simulink model "Gate_Harness"  (R2022b)
settings: Solver=VariableStepAuto  StartTime=0.0  StopTime=80.0  RelTol=1e-3
(part 1 of 2)
settings Model: Creator=chiar  LastModifiedBy=chiar
settings ConfigComp: CovEnable=on  RecordCoverage=on  CovModelRefEnable=on

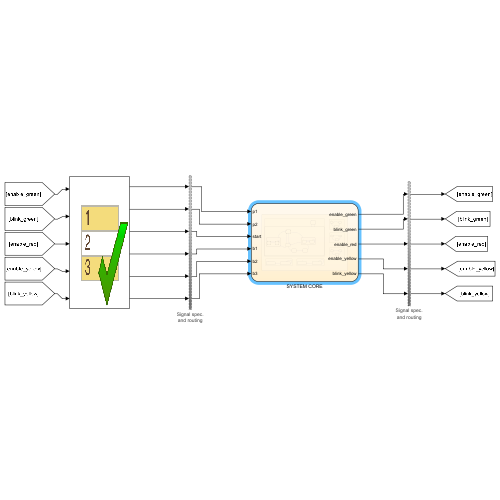
[thumbnail: Simulink's stored preview of the top-level diagram]
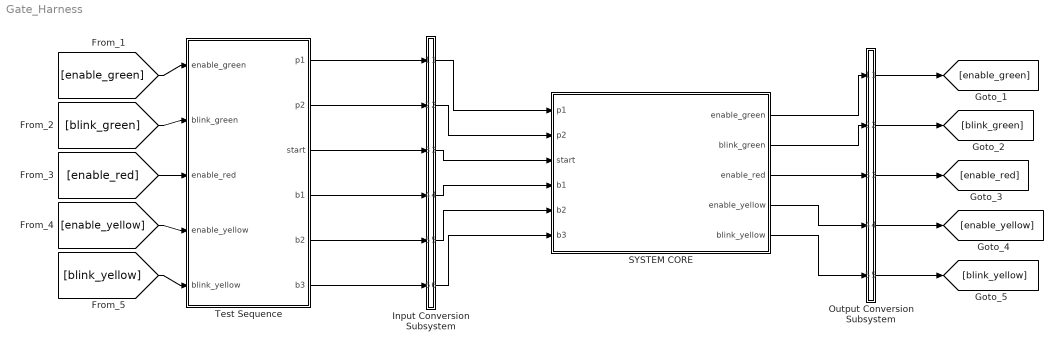
== system Gate_Harness ==
  Input Conversion Subsystem : Subsystem  Tag=__SLT_ICS__  Description=|
      | Signal spec.
      | and routing
      settings: AttributesFormatString=%<Description>
  Output Conversion Subsystem : Subsystem  Tag=__SLT_OCS__  Description=|
      | Signal spec.
      | and routing
      settings: AttributesFormatString=%<Description>
  SYSTEM CORE : Stateflow chart  TreatAsAtomicUnit=on
  Test Sequence : Test Sequence  TreatAsAtomicUnit=on
  wires:
  Test Sequence/1(p1) -> Input Conversion Subsystem/1(Inport_1)
  Test Sequence/2(p2) -> Input Conversion Subsystem/2(Inport_2)
  Test Sequence/3(start) -> Input Conversion Subsystem/3(Inport_3)
  Test Sequence/4(b1) -> Input Conversion Subsystem/4(Inport_4)
  Test Sequence/5(b2) -> Input Conversion Subsystem/5(Inport_5)
  Test Sequence/6(b3) -> Input Conversion Subsystem/6(Inport_6)
  [enable_green] -> Test Sequence/1(enable_green)
  [blink_green] -> Test Sequence/2(blink_green)
  [enable_red] -> Test Sequence/3(enable_red)
  [enable_yellow] -> Test Sequence/4(enable_yellow)
  [blink_yellow] -> Test Sequence/5(blink_yellow)
  Output Conversion Subsystem/1(Outport_1) -> [enable_green]
  Output Conversion Subsystem/2(Outport_2) -> [blink_green]
  Output Conversion Subsystem/3(Outport_3) -> [enable_red]
  Output Conversion Subsystem/4(Outport_4) -> [enable_yellow]
  Output Conversion Subsystem/5(Outport_5) -> [blink_yellow]
  Input Conversion Subsystem/1(Outport_1) -> SYSTEM CORE/1(p1)
  Input Conversion Subsystem/2(Outport_2) -> SYSTEM CORE/2(p2)
  Input Conversion Subsystem/3(Outport_3) -> SYSTEM CORE/3(start)
  Input Conversion Subsystem/4(Outport_4) -> SYSTEM CORE/4(b1)
  Input Conversion Subsystem/5(Outport_5) -> SYSTEM CORE/5(b2)
  Input Conversion Subsystem/6(Outport_6) -> SYSTEM CORE/6(b3)
  SYSTEM CORE/1(enable_green) -> Output Conversion Subsystem/1(Inport_1)
  SYSTEM CORE/2(blink_green) -> Output Conversion Subsystem/2(Inport_2)
  SYSTEM CORE/3(enable_red) -> Output Conversion Subsystem/3(Inport_3)
  SYSTEM CORE/4(enable_yellow) -> Output Conversion Subsystem/4(Inport_4)
  SYSTEM CORE/5(blink_yellow) -> Output Conversion Subsystem/5(Inport_5)

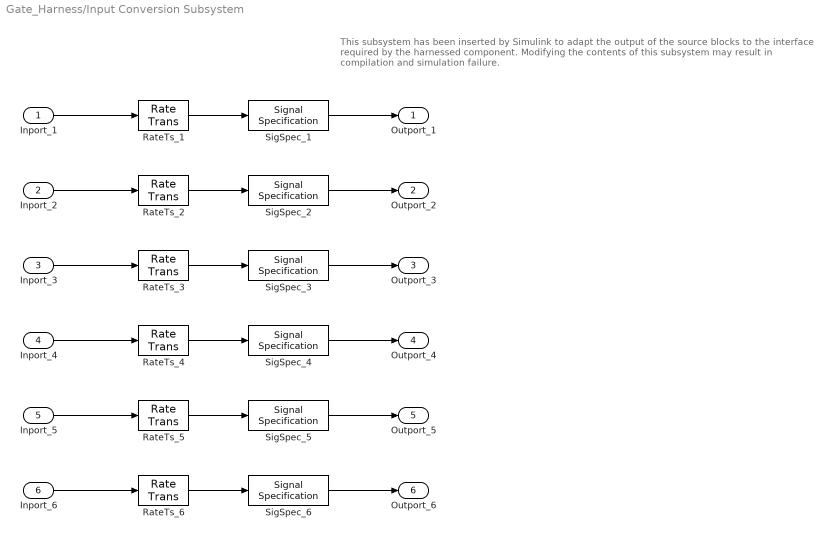
== system Gate_Harness/Input Conversion Subsystem ==
  note: This subsystem has been inserted by Simulink to adapt the output of the source blocks to the interface required by the harnessed component.
      |  Modifying the contents of this subsystem may result in compilation and simulation failure.
  Inport_1 : Inport
  Inport_2 : Inport  Port=2
  Inport_3 : Inport  Port=3
  Inport_4 : Inport  Port=4
  Inport_5 : Inport  Port=5
  Inport_6 : Inport  Port=6
  RateTs_{1..6} (6 alike) : RateTransition  OutPortSampleTime=[-1, 0]
  SigSpec_{1..6} (6 alike) : SignalSpecification  OutDataTypeStr=boolean  Dimensions=[1]  SampleTime=[-1, 0]
  Outport_1 : Outport
  Outport_2 : Outport  Port=2
  Outport_3 : Outport  Port=3
  Outport_4 : Outport  Port=4
  Outport_5 : Outport  Port=5
  Outport_6 : Outport  Port=6
  wires:
  SigSpec_1/1 -> Outport_1/1
  RateTs_1/1 -> SigSpec_1/1
  Inport_1/1 -> RateTs_1/1
  SigSpec_2/1 -> Outport_2/1
  RateTs_2/1 -> SigSpec_2/1
  Inport_2/1 -> RateTs_2/1
  SigSpec_3/1 -> Outport_3/1
  RateTs_3/1 -> SigSpec_3/1
  Inport_3/1 -> RateTs_3/1
  SigSpec_4/1 -> Outport_4/1
  RateTs_4/1 -> SigSpec_4/1
  Inport_4/1 -> RateTs_4/1
  SigSpec_5/1 -> Outport_5/1
  RateTs_5/1 -> SigSpec_5/1
  Inport_5/1 -> RateTs_5/1
  SigSpec_6/1 -> Outport_6/1
  RateTs_6/1 -> SigSpec_6/1
  Inport_6/1 -> RateTs_6/1

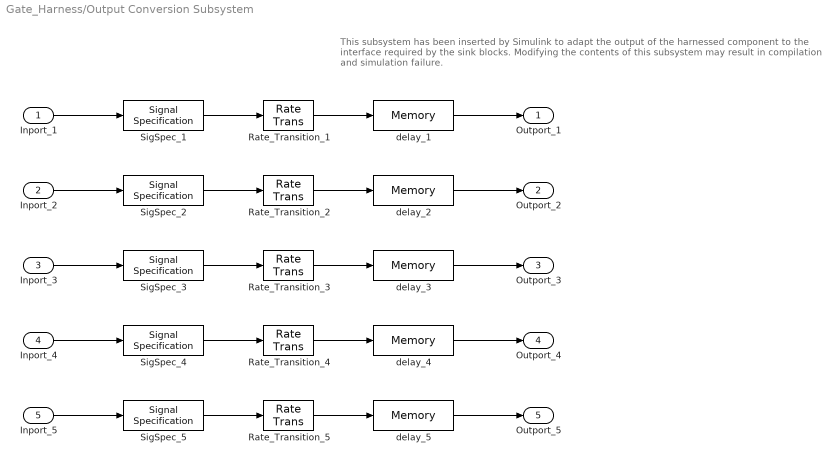
== system Gate_Harness/Output Conversion Subsystem ==
  note: This subsystem has been inserted by Simulink to adapt the output of the harnessed component to the interface required by the sink blocks.
      |  Modifying the contents of this subsystem may result in compilation and simulation failure.
  Inport_1 : Inport
  Inport_2 : Inport  Port=2
  Inport_3 : Inport  Port=3
  Inport_4 : Inport  Port=4
  Inport_5 : Inport  Port=5
  Rate_Transition_{1..5} (5 alike) : RateTransition  OutPortSampleTimeOpt=Inherit
  SigSpec_{1..5} (5 alike) : SignalSpecification  OutDataTypeStr=boolean  Dimensions=[1]
  delay_{1..5} (5 alike) : Memory
  Outport_1 : Outport
  Outport_2 : Outport  Port=2
  Outport_3 : Outport  Port=3
  Outport_4 : Outport  Port=4
  Outport_5 : Outport  Port=5
  wires:
  Inport_1/1 -> SigSpec_1/1
  SigSpec_1/1 -> Rate_Transition_1/1
  Rate_Transition_1/1 -> delay_1/1
  delay_1/1 -> Outport_1/1
  Inport_2/1 -> SigSpec_2/1
  SigSpec_2/1 -> Rate_Transition_2/1
  Rate_Transition_2/1 -> delay_2/1
  delay_2/1 -> Outport_2/1
  Inport_3/1 -> SigSpec_3/1
  SigSpec_3/1 -> Rate_Transition_3/1
  Rate_Transition_3/1 -> delay_3/1
  delay_3/1 -> Outport_3/1
  Inport_4/1 -> SigSpec_4/1
  SigSpec_4/1 -> Rate_Transition_4/1
  Rate_Transition_4/1 -> delay_4/1
  delay_4/1 -> Outport_4/1
  Inport_5/1 -> SigSpec_5/1
  SigSpec_5/1 -> Rate_Transition_5/1
  Rate_Transition_5/1 -> delay_5/1
  delay_5/1 -> Outport_5/1

== stateflow chart Gate_Harness/SYSTEM CORE ==
  state SYSTEM
    state GATE [parallel]
      settings: executionOrder=3
      state INACTIVE
        en:
        enable_green = OFF;
        enable_yellow = OFF;
        enable_red = OFF;
        blink_green = OFF;
        blink_yellow = OFF;
      state ACTIVE
        state IS_OPENING
          en:
          enable_red = OFF;
          enable_yellow=OFF;
          enable_green=OFF;
          blink_green = OFF;
          blink_yellow = ON;
        state OPEN
          state GREEN_BLK_OFF
            en:
            enable_green = ON;
            enable_red = ON;
            enable_yellow = ON;
            blink_green = OFF;
            blink_yellow = OFF;
          state GREEN_BLK_ON
            en:
            enable_green = OFF;
            enable_red = OFF;
            enable_yellow = OFF;
            blink_green = ON;
            blink_yellow = OFF;
          (default) -> SYSTEM.GATE.ACTIVE.OPEN.GREEN_BLK_OFF
          SYSTEM.GATE.ACTIVE.OPEN.GREEN_BLK_ON -> SYSTEM.GATE.ACTIVE.OPEN.GREEN_BLK_ON [order 2] : [b1_pressed & (p1 == OFF)]
          SYSTEM.GATE.ACTIVE.OPEN.GREEN_BLK_OFF -> SYSTEM.GATE.ACTIVE.OPEN.GREEN_BLK_ON : [b1_pressed & (p1 == OFF)]
          SYSTEM.GATE.ACTIVE.OPEN.GREEN_BLK_ON -> SYSTEM.GATE.ACTIVE.OPEN.GREEN_BLK_OFF [order 1] : [after(GREENDUR, sec) | (p1 == ON)]
        state CLOSE
          state GREEN_BLK_OFF
            en:
            enable_green = OFF;
            enable_red = OFF;
            enable_yellow = OFF;
            blink_green = OFF;
            blink_yellow = OFF;
          state GREEN_BLK_ON
            en:
            enable_green = OFF;
            enable_red = OFF;
            enable_yellow = OFF;
            blink_green = ON;
            blink_yellow = OFF;
          (default) -> SYSTEM.GATE.ACTIVE.CLOSE.GREEN_BLK_OFF
          SYSTEM.GATE.ACTIVE.CLOSE.GREEN_BLK_ON -> SYSTEM.GATE.ACTIVE.CLOSE.GREEN_BLK_ON [order 2] : [b1_pressed & (p1 == OFF)]
          SYSTEM.GATE.ACTIVE.CLOSE.GREEN_BLK_OFF -> SYSTEM.GATE.ACTIVE.CLOSE.GREEN_BLK_ON : [b1_pressed & (p1 == OFF)]
          SYSTEM.GATE.ACTIVE.CLOSE.GREEN_BLK_ON -> SYSTEM.GATE.ACTIVE.CLOSE.GREEN_BLK_OFF [order 1] : [after(GREENDUR, sec) | (p1 == ON)]
        state IS_CLOSING
          en:
          enable_red = OFF;
          enable_yellow=OFF;
          enable_green=OFF;
          blink_green = OFF;
          blink_yellow = ON;
        note: Per i sensori stiamo usando la logica negata.
        state STOP_SYSTEM
          en:
          enable_red = OFF;
          enable_yellow=OFF;
          enable_green=OFF;
          blink_green = OFF;
          blink_yellow = OFF;
        state ERROR_STATE
          en:
          enable_red = ON;
          enable_yellow=OFF;
          enable_green=OFF;
          blink_green = OFF;
          blink_yellow = OFF;
        IS_OPENING -> OPEN [order 2] : after(working_time, sec)
        CLOSE -> IS_OPENING : [b1_pressed & (p1 == ON)]
        IS_CLOSING -> IS_OPENING [order 1] : [b1_pressed | (p1 == OFF)]
        IS_OPENING -> IS_CLOSING [order 1] : [b1_pressed & (p1 == ON)]
        IS_CLOSING -> CLOSE [order 2] : [(p2 == OFF)]
        (default) -> IS_CLOSING
        ERROR_STATE -> CLOSE : [p2 == OFF]
        OPEN -> IS_CLOSING : [(b1_pressed & p1 == ON) | duration(p1 == ON) >= closing_time]
        IS_CLOSING -> STOP_SYSTEM [order 3] : [after(working_time, sec) & (p2 == ON)]
        STOP_SYSTEM -> ERROR_STATE : after(WAITING_TIME,sec)
      (default) -> INACTIVE
      INACTIVE -> ACTIVE : [start == ON]
      ACTIVE -> INACTIVE : [start == OFF]
    state B1 [parallel]
      settings: executionOrder=6
      state RELEASED
      state PRESSED
      state LONG_PRESSED
        send(b1_pressed)
      (default) -> SYSTEM.B1.RELEASED
      SYSTEM.B1.RELEASED -> SYSTEM.B1.PRESSED : [b1==ON]
      SYSTEM.B1.LONG_PRESSED -> SYSTEM.B1.RELEASED : [b1 == OFF]
      SYSTEM.B1.PRESSED -> SYSTEM.B1.LONG_PRESSED : [b1 == OFF]
    state B2 [parallel]
      settings: executionOrder=5
      state RELEASED
      state PRESSED
      state LONG_PRESSED
        send(b2_pressed)
      (default) -> SYSTEM.B2.RELEASED
      SYSTEM.B2.RELEASED -> SYSTEM.B2.PRESSED : [b2==ON]
      SYSTEM.B2.LONG_PRESSED -> SYSTEM.B2.RELEASED : [b2 == OFF]
      SYSTEM.B2.PRESSED -> SYSTEM.B2.LONG_PRESSED : [b2 == OFF]
    state B3 [parallel]
      settings: executionOrder=4
      state RELEASED
      state PRESSED
      state LONG_PRESSED
        send(b3_pressed)
      (default) -> SYSTEM.B3.RELEASED
      SYSTEM.B3.RELEASED -> SYSTEM.B3.PRESSED : [b3==ON]
      SYSTEM.B3.LONG_PRESSED -> SYSTEM.B3.RELEASED : [b3 == OFF]
      SYSTEM.B3.PRESSED -> SYSTEM.B3.LONG_PRESSED : [b3 == OFF]
    state WORKING_TIME [parallel]
      settings: executionOrder=1
      state WORKING_TIME_RESET
        en:
        working_time = 10;
      state WORKING_TIME_INC
        en:
        working_time = mod(working_time, MAX) + INCREMENT;
      WORKING_TIME_INC -> WORKING_TIME_INC : [b3_pressed & p2 == OFF]
      (default) -> WORKING_TIME_RESET
      WORKING_TIME_RESET -> WORKING_TIME_INC : [b3_pressed & p2 == OFF]
    state CLOSING_TIME [parallel]
      settings: executionOrder=2
      state CLOSING_TIME_RESET
        en:
        closing_time = 10;
      state CLOSING_TIME_INC
        en:
        closing_time = mod(closing_time, MAX) + INCREMENT;
      CLOSING_TIME_INC -> CLOSING_TIME_INC : [b2_pressed & p2 == OFF]
      (default) -> CLOSING_TIME_RESET
      CLOSING_TIME_RESET -> CLOSING_TIME_INC : [b2_pressed & p2 == OFF]
  data: GREENDUR constant double =30; WAITING_TIME constant double =10; ON constant boolean =1; OFF constant boolean =0; working_time local double =10; INCREMENT constant double =10; MAX constant double =120; closing_time local double =10; p1 input boolean; p2 input boolean; start input boolean; enable_green output boolean; blink_green output boolean; enable_red output boolean; enable_yellow output boolean; blink_yellow output boolean; b1 input boolean; b2 input boolean; b3 input boolean
  events: b3_pressed local RISING_EDGE_EVENT; b1_pressed local RISING_EDGE_EVENT; b2_pressed local RISING_EDGE_EVENT
